simulink model "model_base"  (R2017b)
settings: Solver=VariableStepAuto  StartTime=0.0  StopTime=tfinal  MaxStep=0.1  RelTol=1e-9
values from neighbouring files (symbols this model uses):
  a = param.a    [EOM.m]    (also in KF_EOM.m; parameters.m = 1.08; roadPreview.m = obj.param.a; steadyState_EOM.m)
  a1 = obj.param.a1    [MPC.m]    (also in MPC_constraint.m = 0; RMPC.m; parameters.m = 0)
  a2 = obj.param.a2    [MPC.m]    (also in MPC_constraint.m = 1800; RMPC.m; parameters.m = 1800)
  a3 = obj.param.a3    [MPC.m]    (also in MPC_constraint.m = 100; RMPC.m; parameters.m = 100)
  a4 = obj.param.a4    [MPC.m]    (also in MPC_constraint.m = -100; RMPC.m; parameters.m = -100)
  a5 = obj.param.a5    [MPC.m]    (also in MPC_constraint.m = -1800; RMPC.m; parameters.m = -1800)
  A_road = sqrt(2*P*Dn)    [parameters.m]    (also in roadPreview.m = obj.param.A_road)
  b = param.b    [EOM.m]    (also in KF_EOM.m; parameters.m = 1.35; roadPreview.m = obj.param.b; spring.m = [0 (-ones(1,2*ne)).^j 0])
  B = param.B    [EOM.m]    (also in KF_EOM.m; MPC_EOM.m; RMPC.m = obj.param.B; parameters.m = 7.1)
  b1 = obj.param.b1    [MPC.m]    (also in MPC_constraint.m = 7500; RMPC.m; parameters.m = 7500)
  b2 = obj.param.b2    [MPC.m]    (also in MPC_constraint.m = 3000; RMPC.m; parameters.m = 3000)
  b3 = obj.param.b3    [MPC.m]    (also in MPC_constraint.m = 1666.66666667; RMPC.m; parameters.m = 1666.66666667)
  b4 = obj.param.b4    [MPC.m]    (also in MPC_constraint.m = 1666.66666667; RMPC.m; parameters.m = 1666.66666667)
  b5 = obj.param.b5    [MPC.m]    (also in MPC_constraint.m = 3000; RMPC.m; parameters.m = 3000)
  bcF = 2*zetac*omegasF*mF    (= 0)    [parameters.m]
  bcR = 2*zetac*omegasR*mR    (= 0)    [parameters.m]
  brake_init = [0; 0; 0; 0; x0]    [main.m]
  bsF = param.bsF    [EOM.m]    (also in KF_EOM.m; parameters.m = 3825.76172037; steadyState_EOM.m)
  bsR = param.bsR    [EOM.m]    (also in KF_EOM.m; parameters.m = 3672.73125156; steadyState_EOM.m)
  bt = param.bt    [EOM.m]    (also in KF_EOM.m; parameters.m = 0; steadyState_EOM.m)
  C = param.C    [EOM.m]    (also in KF_EOM.m; MPC_EOM.m; RMPC.m = obj.param.C; buildRoadFromPSD.m = 1e-06)
  Ccal = 1/kcal    (= 2.98507462687e-08)    [parameters.m]
  Ccyl = V0_brake/bhf    (= 1.88235294118e-14)    [parameters.m]
  D = param.D    [EOM.m]    (also in KF_EOM.m; MPC_EOM.m; RMPC.m = obj.param.D; parameters.m = 0.5)
  d_bump = 5    [parameters.m]    (also in roadPreview.m = obj.param.d_bump)
  g = param.g    [EOM.m]    (also in KF_EOM.m; MPC_EOM.m; RMPC.m = obj.param.g; parameters.m = 9.81)
  GcF_noInt = minreal(tf('s')*GcF)    [main.m]
  GcR_noInt = minreal(tf('s')*GcR)    [main.m]
  h_susp = param.h_susp    [EOM.m]    (also in KF_EOM.m; parameters.m = 0.2; steadyState_EOM.m)
  Icyl = mcyl    (= 0.75)    [parameters.m]
  Iline = phf*lline/(pi*dline^2/4)    (= 294259805.894)    [parameters.m]
  J = param.J    [EOM.m]    (also in KF_EOM.m; parameters.m = 1398.222; steadyState_EOM.m)
  Jw = param.Jw    [EOM.m]    (also in KF_EOM.m; MPC_EOM.m; RMPC.m = obj.param.Jw; parameters.m = 0.9)
  kcal = 3.35e7    (= 33500000)    [parameters.m]
  ksF = param.ksF    [EOM.m]    (also in KF_EOM.m; parameters.m = 30047.4622878; steadyState_EOM.m)
  ksR = param.ksR    [EOM.m]    (also in KF_EOM.m; parameters.m = 34614.6765555; steadyState_EOM.m)
  kt = param.kt    [EOM.m]    (also in KF_EOM.m; MPC_EOM.m; RMPC.m = obj.param.kt; parameters.m = 355305.758439)
  lambda_road = 50/3.6    (= 13.8888888889)    [parameters.m]    (also in roadPreview.m = obj.param.lambda_road)
  m = param.m    [EOM.m]    (also in KF_EOM.m; RMPC.m = [-ulb; uub]; parameters.m = 1370; steadyState_EOM.m)
  mF = param.mF    [EOM.m]    (also in KF_EOM.m; parameters.m = 761.111111111; steadyState_EOM.m)
  mR = param.mR    [EOM.m]    (also in KF_EOM.m; parameters.m = 608.888888889; steadyState_EOM.m)
  mucal = 0.4    [parameters.m]
  mus = param.mus    [EOM.m]    (also in KF_EOM.m; MPC.m = obj.param.mus; MPC_EOM.m; MPC_constraint.m)
  n_road = nmin:Dn:nmax    [parameters.m]    (also in roadPreview.m = obj.param.n_road)
  Phase_road = 2*pi*rand(size(A_road))    [parameters.m]    (also in roadPreview.m = obj.param.Phase_road)
  Rcyl = bcyl    (= 2500)    [parameters.m]
  reff = 0.112    [parameters.m]
  Rline = 128*phf*vhf*lline/(pi*dline^4)    (= 31387712628.7)    [parameters.m]
  roadProfile_index = 3    [getRoadIndex.m]    (also in main.m = getRoadIndex(roadProfile_name); roadPreview.m = obj.param.roadProfile_index)
  rw = param.rw    [EOM.m]    (also in KF_EOM.m; MPC_EOM.m; RMPC.m = obj.param.rw; parameters.m = 0.3)
  SAcyl = pi*dcyl^2/4    (= 0.00255175863288)    [parameters.m]
  state_init = [0 ... (first row only)    [main.m]
  sx_ref = -0.3    [MPC.m]    (also in RMPC.m; main.m = -1/B*tan(pi/(2*C)))
  sxABSoff = 0.1*sx_ref    [main.m]
  sxABSon_F = 1.4*sx_ref    [main.m]
  torque_request = -3000    [main.m]
  Ts_MPC = 0.05    [main.m]    (also in roadPreview.m = 0.01)
  U_cutoff = 10/3.6    (= 2.77777777778)    [main.m]
  w_road = 2*2*pi/lambda_road    (= 0.904778684234)    [parameters.m]    (also in roadPreview.m = obj.param.w_road)
  x0 = 0.00015    [parameters.m]    (also in test_minmaxMPC.m = rand(Nx,1))
  z0_road = 0.03    [parameters.m]    (also in roadPreview.m = obj.param.z0_road)
libraries: simulink x1
settings Model: Creator=louis  LastModifiedBy=louis

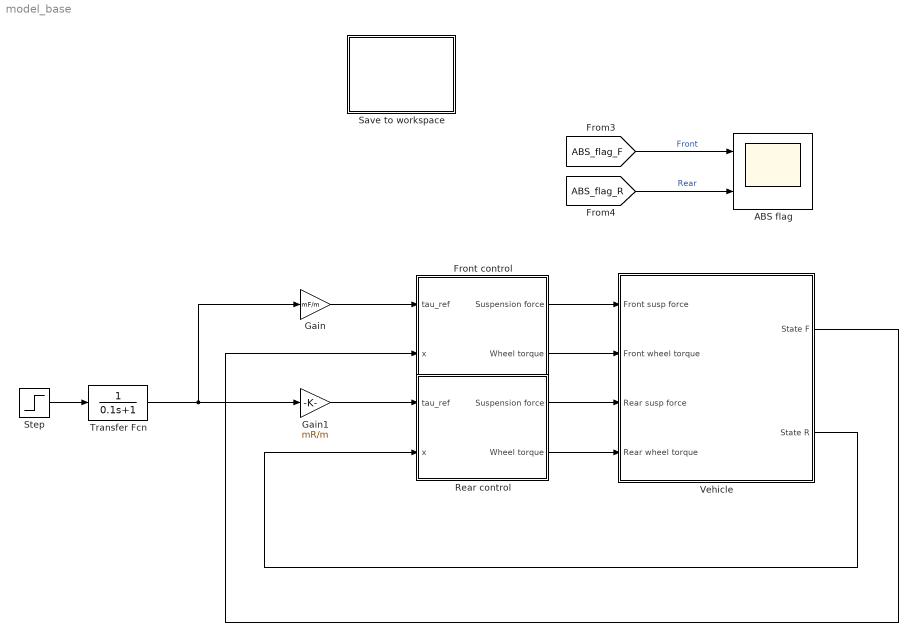
== system model_base ==
  ABS flag : Scope  NumInputPorts=2
  Front control : Subsystem
  Gain : Gain  Gain=mF/m
  Gain1 : Gain  Gain=mR/m
  Rear control : Subsystem
  Save to workspace : Subsystem
  Step : Step  After=torque_request  SampleTime=0
  Transfer Fcn : TransferFcn  Denominator=[0.1 1]
  Vehicle : Subsystem
  wires:
  Step/1 -> Transfer Fcn/1
  Transfer Fcn/1 -> Gain/1, Gain1/1
  Rear control/2(Wheel torque) -> Vehicle/4(Rear wheel torque)
  Vehicle/1(State F) -> Front control/2(x)
  Vehicle/2(State R) -> Rear control/2(x)
  Front control/2(Wheel torque) -> Vehicle/2(Front wheel torque)
  [ABS_flag_F] -> ABS flag/1  "Front"
  [ABS_flag_R] -> ABS flag/2  "Rear"
  Gain/1 -> Front control/1(tau_ref)
  Gain1/1 -> Rear control/1(tau_ref)
  Rear control/1(Suspension force) -> Vehicle/3(Rear susp force)
  Front control/1(Suspension force) -> Vehicle/1(Front susp force)

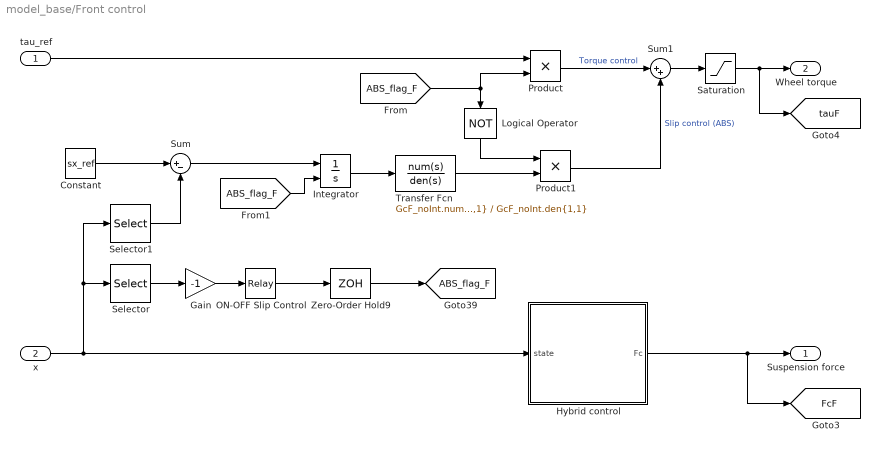
== system model_base/Front control ==
  tau_ref : Inport
  x : Inport  Port=2
  Constant : Constant  Value=sx_ref
  Gain : Gain  Gain=-1
  Hybrid control : MATLAB Function  TreatAsAtomicUnit=on
  Integrator : Integrator  ExternalReset=rising
  Logical Operator : Logic  Operator=NOT  AllPortsSameDT=off  OutDataTypeStr=boolean
  ON-OFF Slip Control : Relay  OnSwitchValue=-sxABSon_F  OffSwitchValue=-sxABSoff  OnOutputValue=0  OffOutputValue=1
  Product : Product
  Product1 : Product
  Saturation : Saturate  UpperLimit=0  LowerLimit=-Inf
  Selector : Selector  IndexOptions=Index vector (dialog)  Indices=5  OutputSizes=1
  Selector1 : Selector  IndexOptions=Index vector (dialog)  Indices=5  OutputSizes=1
  Sum : Sum  Inputs=|+-
  Sum1 : Sum  Inputs=|++
  Transfer Fcn : TransferFcn  Numerator=GcF_noInt.num{1,1}  Denominator=GcF_noInt.den{1,1}
  Zero-Order Hold9 : ZeroOrderHold  SampleTime=Ts_MPC
  Suspension force : Outport
  Wheel torque : Outport  Port=2
  tag scope: ABS_flag_F=global, FcF=global, tauF=global
  wires:
  x/1 -> Hybrid control/1(state), Selector1/1, Selector/1
  Zero-Order Hold9/1 -> [ABS_flag_F]
  Gain/1 -> ON-OFF Slip Control/1
  Selector/1 -> Gain/1
  ON-OFF Slip Control/1 -> Zero-Order Hold9/1
  tau_ref/1 -> Product/1
  Sum1/1 -> Saturation/1
  Hybrid control/1(Fc) -> [FcF], Suspension force/1
  Integrator/1 -> Transfer Fcn/1
  [ABS_flag_F] -> Product/2, Logical Operator/1
  Logical Operator/1 -> Product1/1
  Constant/1 -> Sum/1
  Transfer Fcn/1 -> Product1/2
  [ABS_flag_F] -> Integrator/2
  Sum/1 -> Integrator/1
  Selector1/1 -> Sum/2
  Product/1 -> Sum1/1  "Torque control"
  Product1/1 -> Sum1/2  "Slip control (ABS)"
  Saturation/1 -> [tauF], Wheel torque/1

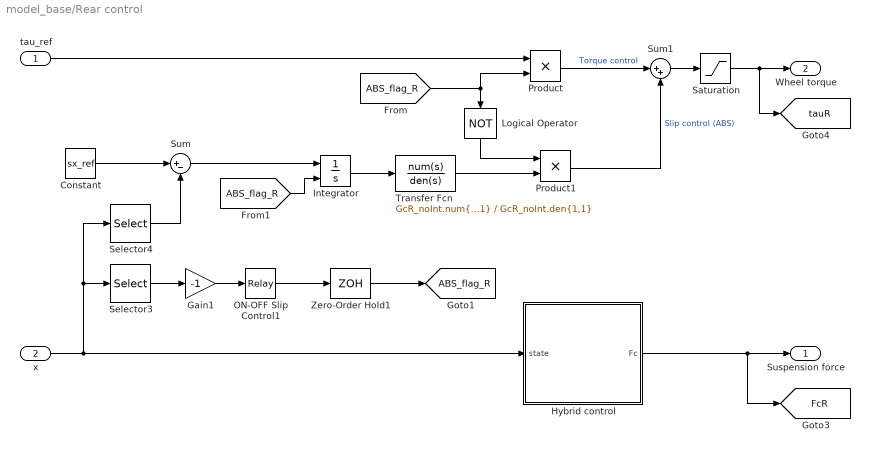
== system model_base/Rear control ==
  tau_ref : Inport
  x : Inport  Port=2
  Constant : Constant  Value=sx_ref
  Gain1 : Gain  Gain=-1
  Hybrid control : MATLAB Function  TreatAsAtomicUnit=on
  Integrator : Integrator  ExternalReset=either
  Logical Operator : Logic  Operator=NOT  AllPortsSameDT=off  OutDataTypeStr=boolean
  ON-OFF Slip Control1 : Relay  OnSwitchValue=-sxABSon_F  OffSwitchValue=-sxABSoff  OnOutputValue=0  OffOutputValue=1
  Product : Product
  Product1 : Product
  Saturation : Saturate  UpperLimit=0  LowerLimit=-Inf
  Selector3 : Selector  IndexOptions=Index vector (dialog)  Indices=5  OutputSizes=1
  Selector4 : Selector  IndexOptions=Index vector (dialog)  Indices=5  OutputSizes=1
  Sum : Sum  Inputs=|+-
  Sum1 : Sum  Inputs=|++
  Transfer Fcn : TransferFcn  Numerator=GcR_noInt.num{1,1}  Denominator=GcR_noInt.den{1,1}
  Zero-Order Hold1 : ZeroOrderHold  SampleTime=Ts_MPC
  Suspension force : Outport
  Wheel torque : Outport  Port=2
  tag scope: ABS_flag_R=global, FcR=global, tauR=global
  wires:
  ON-OFF Slip Control1/1 -> Zero-Order Hold1/1
  Selector3/1 -> Gain1/1
  Zero-Order Hold1/1 -> [ABS_flag_R]
  Sum1/1 -> Saturation/1
  tau_ref/1 -> Product/1
  Product1/1 -> Sum1/2  "Slip control (ABS)"
  Gain1/1 -> ON-OFF Slip Control1/1
  Logical Operator/1 -> Product1/1
  [ABS_flag_R] -> Integrator/2
  Constant/1 -> Sum/1
  Hybrid control/1(Fc) -> [FcR], Suspension force/1
  Product/1 -> Sum1/1  "Torque control"
  Integrator/1 -> Transfer Fcn/1
  [ABS_flag_R] -> Product/2, Logical Operator/1
  Selector4/1 -> Sum/2
  x/1 -> Hybrid control/1(state), Selector4/1, Selector3/1
  Sum/1 -> Integrator/1
  Transfer Fcn/1 -> Product1/2
  Saturation/1 -> [tauR], Wheel torque/1

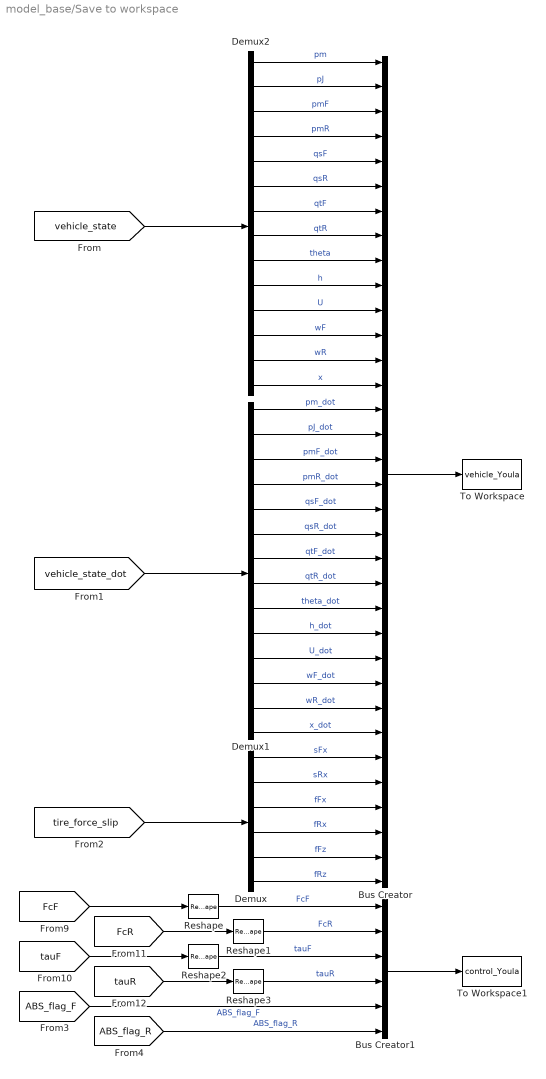
== system model_base/Save to workspace ==
  Bus Creator : BusCreator  Inputs=34
  Bus Creator1 : BusCreator  Inputs=6
  Demux : Demux  Outputs=6
  Demux1 : Demux  Outputs=14
  Demux2 : Demux  Outputs=14
  Reshape{,1..3} (4 alike) : Reshape
  To Workspace : ToWorkspace  VariableName=vehicle_Youla  SaveFormat=Timeseries  SampleTime=-1
  To Workspace1 : ToWorkspace  VariableName=control_Youla  SaveFormat=Timeseries  SampleTime=-1
  wires:
  Demux/1 -> Bus Creator/29  "sFx"
  [tire_force_slip] -> Demux/1
  Demux/2 -> Bus Creator/30  "sRx"
  Demux/3 -> Bus Creator/31  "fFx"
  Demux/5 -> Bus Creator/33  "fFz"
  [vehicle_state] -> Demux2/1
  Bus Creator/1 -> To Workspace/1
  Demux2/1 -> Bus Creator/1  "pm"
  Demux2/2 -> Bus Creator/2  "pJ"
  Demux2/3 -> Bus Creator/3  "pmF"
  Demux2/4 -> Bus Creator/4  "pmR"
  Demux2/5 -> Bus Creator/5  "qsF"
  Demux2/6 -> Bus Creator/6  "qsR"
  Demux2/7 -> Bus Creator/7  "qtF"
  Demux2/8 -> Bus Creator/8  "qtR"
  Demux2/9 -> Bus Creator/9  "theta"
  Demux2/11 -> Bus Creator/11  "U"
  Demux2/12 -> Bus Creator/12  "wF"
  Demux2/13 -> Bus Creator/13  "wR"
  Demux2/14 -> Bus Creator/14  "x"
  Demux/6 -> Bus Creator/34  "fRz"
  Demux/4 -> Bus Creator/32  "fRx"
  Demux1/2 -> Bus Creator/16  "pJ_dot"
  Demux1/11 -> Bus Creator/25  "U_dot"
  Demux1/8 -> Bus Creator/22  "qtR_dot"
  Demux1/4 -> Bus Creator/18  "pmR_dot"
  Demux1/5 -> Bus Creator/19  "qsF_dot"
  Demux1/9 -> Bus Creator/23  "theta_dot"
  Demux1/14 -> Bus Creator/28  "x_dot"
  Demux1/1 -> Bus Creator/15  "pm_dot"
  Demux1/13 -> Bus Creator/27  "wR_dot"
  Demux1/7 -> Bus Creator/21  "qtF_dot"
  [vehicle_state_dot] -> Demux1/1
  Demux1/3 -> Bus Creator/17  "pmF_dot"
  Demux1/12 -> Bus Creator/26  "wF_dot"
  Demux1/6 -> Bus Creator/20  "qsR_dot"
  Demux2/10 -> Bus Creator/10  "h"
  Demux1/10 -> Bus Creator/24  "h_dot"
  [ABS_flag_F] -> Bus Creator1/5  "ABS_flag_F"
  [ABS_flag_R] -> Bus Creator1/6  "ABS_flag_R"
  Bus Creator1/1 -> To Workspace1/1
  Reshape1/1 -> Bus Creator1/2  "FcR"
  Reshape/1 -> Bus Creator1/1  "FcF"
  Reshape3/1 -> Bus Creator1/4  "tauR"
  Reshape2/1 -> Bus Creator1/3  "tauF"
  [FcF] -> Reshape/1
  [FcR] -> Reshape1/1
  [tauF] -> Reshape2/1
  [tauR] -> Reshape3/1

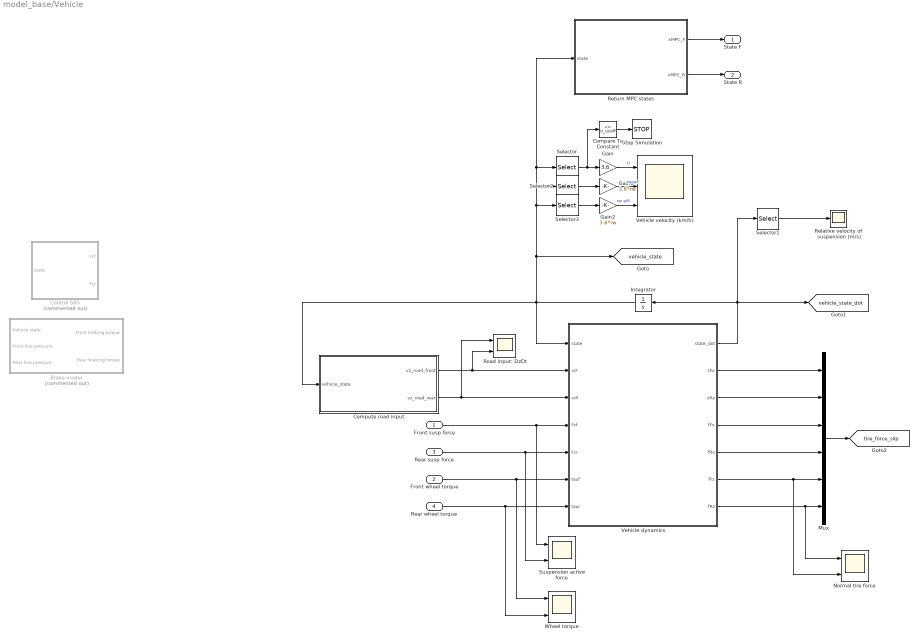
== system model_base/Vehicle ==
  Front susp force : Inport
  Front wheel torque : Inport  Port=2
  Rear susp force : Inport  Port=3
  Rear wheel torque : Inport  Port=4
  Brake model : Subsystem  Commented=on
  Compare To Constant : simulink/Logic and Bit Operations/Compare To Constant  relop=<=  const=U_cutoff  OutDataTypeStr=boolean
  Compute road input : MATLAB Function  TreatAsAtomicUnit=on
  Control SAS : MATLAB Function  Commented=on  TreatAsAtomicUnit=on
  Gain : Gain  Gain=3.6
  Gain1 : Gain  Gain=3.6*rw
  Gain2 : Gain  Gain=3.6*rw
  Integrator : Integrator  InitialCondition=state_init
  Mux : Mux  Inputs=6
  Normal tire force : Scope  NumInputPorts=2
  Relative velocity of suspension (m/s) : Scope
  Return MPC states : MATLAB Function  TreatAsAtomicUnit=on
  Road input: DzDt : Scope  NumInputPorts=2
  Selector : Selector  IndexOptions=Index vector (dialog)  Indices=11  OutputSizes=1
  Selector1 : Selector  IndexOptions=Index vector (dialog)  Indices=[5 6]  OutputSizes=1
  Selector2 : Selector  IndexOptions=Index vector (dialog)  Indices=12  OutputSizes=1
  Selector3 : Selector  IndexOptions=Index vector (dialog)  Indices=13  OutputSizes=1
  Stop Simulation : Stop
  Suspension active force : Scope  NumInputPorts=2
  Vehicle dynamics : MATLAB Function  TreatAsAtomicUnit=on
  Vehicle velocity (km/h) : Scope  NumInputPorts=3
  Wheel torque : Scope  NumInputPorts=2
  State F : Outport
  State R : Outport  Port=2
  tag scope: tire_force_slip=global, vehicle_state=global, vehicle_state_dot=global
  wires:
  Gain/1 -> Vehicle velocity (km/h)/1  "U"
  Vehicle dynamics/7(fRz) -> Normal tire force/1, Mux/6
  Vehicle dynamics/3(sRx) -> Mux/2
  Vehicle dynamics/4(fFx) -> Mux/3
  Vehicle dynamics/5(fRx) -> Mux/4
  Selector/1 -> Compare To Constant/1, Gain/1
  Vehicle dynamics/2(sFx) -> Mux/1
  Vehicle dynamics/1(state_dot) -> Integrator/1, Selector1/1, [vehicle_state_dot]
  Vehicle dynamics/6(fFz) -> Normal tire force/2, Mux/5
  Mux/1 -> [tire_force_slip]
  Compute road input/2(vz_road_rear) -> Vehicle dynamics/3(viR), Road input: DzDt/1
  Front wheel torque/1 -> Wheel torque/1, Vehicle dynamics/6(tauf)
  Rear wheel torque/1 -> Wheel torque/2, Vehicle dynamics/7(taur)
  Compare To Constant/1 -> Stop Simulation/1
  Front susp force/1 -> Suspension active force/1, Vehicle dynamics/4(Fcf)
  Rear susp force/1 -> Suspension active force/2, Vehicle dynamics/5(Fcr)
  Compute road input/1(vz_road_front) -> Vehicle dynamics/2(viF), Road input: DzDt/2
  Selector1/1 -> Relative velocity of suspension (m/s)/1
  Integrator/1 -> Vehicle dynamics/1(state), [vehicle_state], Selector3/1, Selector2/1, Return MPC states/1(state), Selector/1, Compute road input/1(vehicle_state)
  Return MPC states/1(xMPC_F) -> State F/1
  Return MPC states/2(xMPC_R) -> State R/1
  Selector2/1 -> Gain1/1
  Gain1/1 -> Vehicle velocity (km/h)/2  "rw wF"
  Gain2/1 -> Vehicle velocity (km/h)/3  "rw wR"
  Selector3/1 -> Gain2/1

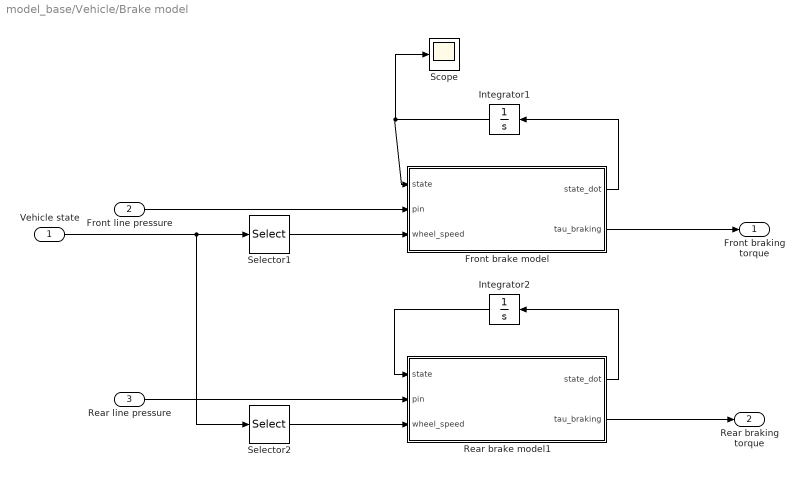
== system model_base/Vehicle/Brake model ==
  Vehicle state : Inport
  Front line pressure : Inport  Port=2
  Rear line pressure : Inport  Port=3
  Front brake model : MATLAB Function  TreatAsAtomicUnit=on
  Integrator1 : Integrator  InitialCondition=brake_init
  Integrator2 : Integrator  InitialCondition=brake_init
  Rear brake model1 : MATLAB Function  TreatAsAtomicUnit=on
  Scope : Scope
  Selector1 : Selector  IndexOptions=Index vector (dialog)  Indices=12  OutputSizes=1
  Selector2 : Selector  IndexOptions=Index vector (dialog)  Indices=13  OutputSizes=1
  Front braking torque : Outport
  Rear braking torque : Outport  Port=2
  wires:
  Front brake model/1(state_dot) -> Integrator1/1
  Vehicle state/1 -> Selector2/1, Selector1/1
  Integrator1/1 -> Scope/1, Front brake model/1(state)
  Front brake model/2(tau_braking) -> Front braking torque/1
  Selector1/1 -> Front brake model/3(wheel_speed)
  Front line pressure/1 -> Front brake model/2(pin)
  Selector2/1 -> Rear brake model1/3(wheel_speed)
  Rear line pressure/1 -> Rear brake model1/2(pin)
  Integrator2/1 -> Rear brake model1/1(state)
  Rear brake model1/1(state_dot) -> Integrator2/1
  Rear brake model1/2(tau_braking) -> Rear braking torque/1

== matlab function model_base/Vehicle/Compute road input ==
  data: vz_road_front output; vehicle_state input; vz_road_rear output; a parameter; b parameter; J parameter; z0_road parameter; w_road parameter; lambda_road parameter; d_bump parameter; A_road parameter; Phase_road parameter; n_road parameter; roadProfile_index parameter
function [vz_road_front,vz_road_rear] = roadInput(vehicle_state, ...
    a, b, J, z0_road, w_road, lambda_road, d_bump,...
    A_road, Phase_road, n_road, roadProfile_index)

pJ    = vehicle_state(2);
theta = vehicle_state(9);
U     = vehicle_state(11);
x     = vehicle_state(14);
theta_dot = pJ/J;
x_dot     = U;

% Compute longitudinal speed at front and rear wheel
x_front = x + a*cos(theta);
x_rear  = x - b*cos(theta);
DxDt_front = x_dot - a*theta_dot*sin(theta);
DxDt_rear  = x_dot + b*theta_dot*sin(theta);

% Road input at the front wheel is:
% x_dot - a*theta_dot*sin(theta) * dz_road/dx(x -b cos(theta))
DzDx_front = roadProfile(x_front,z0_road,lambda_road,w_road,d_bump,...
    A_road,Phase_road,n_road,roadProfile_index);
vz_road_front = DxDt_front * DzDx_front;

% Road input at the rear wheel is:
% x_dot + b*theta_dot*sin(theta) * dz_road/dx(x -b cos(theta))
DzDx_rear = roadProfile(x_rear,z0_road,lambda_road,w_road,d_bump,...
    A_road,Phase_road,n_road,roadProfile_index);
vz_road_rear = DxDt_rear * DzDx_rear;

== matlab function model_base/Vehicle/Vehicle dynamics ==
  data: state input; viF input; state_dot output; sFx output; sRx output; fFx output; fRx output; fFz output; fRz output; viR input; Fcf input; Fcr input; tauf input; taur input; m parameter; J parameter; a parameter; b parameter; ksR parameter; ksF parameter; bsR parameter; bsF parameter; kt parameter; bt parameter; mus parameter; rw parameter; B parameter; C parameter; D parameter; Jw parameter; g parameter; h_susp parameter; mF parameter; mR parameter
function [state_dot,sFx,sRx,fFx,fRx,fFz,fRz] = ...
    chassisModel(state,viF,viR,Fcf, Fcr,tauf,taur,...
    m, J, a, b, ksR, ksF, bsR, bsF, kt, bt, mus, rw, B, C, D, Jw, g, ...
    h_susp, mF, mR)

%% Rename state variables
% Vertical dynamics
pm    = state(1);
pJ    = state(2);
pmF   = state(3);
pmR   = state(4);
qsF   = state(5);
qsR   = state(6);
qtF   = state(7);
qtR   = state(8);
theta = state(9);
% h     = state(10);
% Longitudinal dynamics
U     = state(11);
wF    = state(12);
wR    = state(13);
% x     = state(14);

% Compute vertical velocities at the front and rear of the sprung mass
vR  = pm/m - b*cos(theta) * pJ/J;
vF  = pm/m + a*cos(theta) * pJ/J;

% Compute distance
h_susp_F = h_susp - qsF;            % Height of the front suspension
h_susp_R = h_susp - qsR;            % Height of the rear suspension
rwF_unladen = rw + (mF+mus)*g/kt;   % Unladen front wheel radius
rwR_unladen = rw + (mR+mus)*g/kt;   % Unladen rear wheel radius
rwF = min(rw - qtF, rwF_unladen);   % Front tire radius
rwR = min(rw - qtR, rwR_unladen);   % Rear tire radius

%% Compute suspension and tire forces
% Suspension vertical forces (gauge)
fsF = ksF*qsF + Fcf + bsF*(pmF/mus - vF);
fsR = ksR*qsR + Fcr + bsR*(pmR/mus - vR);

% data = [ -1410, -5008;
%  -720, -3436;
%  -390, -2324;
%  -210, -1792;
%  -90, -1008;
%  -20, -228;
%  20, 228;
%  90, 596;
%  200, 784;
%  390, 1100;
%  760, 1796;
%  1160, 2560];
% v_rel = data(:,1)*1e-3; % Relative velocity (m/s)
% F_damper = 2*data(:,2); % Damper force for one axle (N)
% % TODO check sign: 
% % is it interp1(v_rel,-F_damper,-(pmF/mus - vF),'linear','extrap')
% % or interp1(v_rel,F_damper,(pmF/mus - vF),'linear','extrap')
% F_damper_F = interp1(v_rel,-F_damper,-(pmF/mus - vF),'linear','extrap');
% F_damper_R = interp1(v_rel,-F_damper,-(pmR/mus - vR),'linear','extrap');
% fsF = ksF*qsF + Fcf + F_damper_F;
% fsR = ksR*qsR + Fcr + F_damper_R;

% Tire vertical forces (gauge)
ftF = kt*qtF + bt*(viF - pmF/mus);
ftR = kt*qtR + bt*(viR - pmR/mus);

% Make sure the tire vertical force cannot be negative
ftF = max(-(mus + mF)*g,ftF);
ftR = max(-(mus + mR)*g,ftR);

%% Compute longitudinal tire force
% Compute longitudinal slip ratio
% Front slip ratio
den = max(rwF * wF, U);
if den ~= 0
    sFx = (rwF * wF - U) / den;
else
    sFx = 0;
end
% Rear slip ratio
den = max(rwR * wR, U);
if den ~= 0
    sRx = (rwR * wR - U) / den;
else
    sRx = 0;
end

% Compute friction coefficient (simplified Pacejka's tire model)
muF = D * sin(C * atan(B * sFx));
muR = D * sin(C * atan(B * sRx));

% Compute normal force
fFz = ftF + (mus + mF)*g;
fRz = ftR + (mus + mR)*g;

% Compute longitudinal force
fFx = fFz * muF;
fRx = fRz * muR;


%% Compute the state derivatives
% Vertical dynamics
pm_dot    = fsR + fsF;
pJ_dot    = a*cos(theta) * fsF - b*cos(theta) * fsR ...
          + (h_susp_F + rwF - a*sin(theta)) * fFx ...
          + (h_susp_R + rwR + b*sin(theta)) * fRx;
pmF_dot   = ftF - fsF;
pmR_dot   = ftR - fsR;
qsF_dot   = pmF/mus - vF;
qsR_dot   = pmR/mus - vR;
qtF_dot   = viF - pmF/mus;
qtR_dot   = viR - pmR/mus;
theta_dot = pJ/J;
h_dot     = pm/m;

% Longitudinal dynamics
U_dot = 1/(m+2*mus) * (fFx + fRx);
wF_dot = 1/Jw * (tauf - rwF*fFx);
wR_dot = 1/Jw * (taur - rwR*fRx);
x_dot = U;

%% Return the state derivatives
state_dot = [pm_dot; pJ_dot; pmF_dot; pmR_dot;...
    qsF_dot; qsR_dot; qtF_dot; qtR_dot; theta_dot; h_dot;...
    U_dot; wF_dot; wR_dot; x_dot];

end

== matlab function model_base/Vehicle/Brake model/Front brake model ==
  data: state input; state_dot output; pin input; wheel_speed input; tau_braking output; Icyl parameter; Rcyl parameter; Ccal parameter; Iline parameter; Rline parameter; Ccyl parameter; SAcyl parameter; mucal parameter; kcal parameter; reff parameter; x0 parameter
function [state_dot, tau_braking] = brakeModel(state, pin, wheel_speed, ...
    Icyl, Rcyl, Ccal, Iline, Rline, Ccyl, SAcyl, mucal, kcal, reff, x0)

%% Rename state variables
pline = state(1);
qcyl  = state(2);
pcyl  = state(3);
qcal  = state(4);
xcal  = state(5);

%% Equation of motion
pline_dot = pin - Rline*pline/Iline - qcyl/Ccyl;
qcyl_dot  = pline/Iline - SAcyl*pcyl/Icyl;
pcyl_dot  = SAcyl*qcyl/Ccyl - Rcyl*pcyl/Icyl - qcal/Ccal;
qcal_dot  = pcyl/Icyl;
xcal_dot  = pcyl/Icyl;

%% Pack state derivatives
state_dot = [pline_dot; qcyl_dot; pcyl_dot; qcal_dot; xcal_dot];

%% Compute braking torque
tau_braking = 2*mucal*reff*kcal * max(xcal - x0, 0);
% Braking torque is always in the opposite direction to the wheelspeed
tau_braking = -tau_braking * sign(wheel_speed);

== matlab function model_base/Vehicle/Brake model/Rear brake model1 ==
  data: state input; state_dot output; pin input; wheel_speed input; tau_braking output; Icyl parameter; Rcyl parameter; Ccal parameter; Iline parameter; Rline parameter; Ccyl parameter; SAcyl parameter; mucal parameter; kcal parameter; reff parameter; x0 parameter
function [state_dot, tau_braking] = brakeModel(state, pin, wheel_speed, ...
    Icyl, Rcyl, Ccal, Iline, Rline, Ccyl, SAcyl, mucal, kcal, reff, x0)

%% Rename state variables
pline = state(1);
qcyl  = state(2);
pcyl  = state(3);
qcal  = state(4);
xcal  = state(5);

%% Equation of motion
pline_dot = pin - Rline*pline/Iline - qcyl/Ccyl;
qcyl_dot  = pline/Iline - SAcyl*pcyl/Icyl;
pcyl_dot  = SAcyl*qcyl/Ccyl - Rcyl*pcyl/Icyl - qcal/Ccal;
qcal_dot  = pcyl/Icyl;
xcal_dot  = pcyl/Icyl;

%% Pack state derivatives
state_dot = [pline_dot; qcyl_dot; pcyl_dot; qcal_dot; xcal_dot];

%% Compute braking torque
tau_braking = 2*mucal*reff*kcal * max(xcal - x0, 0);
% Braking torque is always in the opposite direction to the wheelspeed
tau_braking = -tau_braking * sign(wheel_speed);

== matlab function model_base/Vehicle/Control SAS ==
  data: Fcf output; Fcr output; state input; m parameter; a parameter; b parameter; J parameter; bcF parameter; bcR parameter; mus parameter
function [Fcf,Fcr] = controlSAS(state,m, a, b, J, bcF, bcR, mus)

pm    = state(1);
pJ    = state(2);
pmF   = state(3);
pmR   = state(4);
theta = state(9);

vF  = pm/m + a*cos(theta) * pJ/J;
vR  = pm/m - b*cos(theta) * pJ/J;

Fcr = -bcR * vR;
if Fcr * (pmR/mus - vR) < 0
    Fcr = 0;
end
Fcf = -bcF * vF;
if Fcf * (pmF/mus - vF) < 0
    Fcf = 0;
end

== matlab function model_base/Front control/Hybrid control ==
  data: state input; Fc output; mF parameter; mus parameter; a1 parameter; a2 parameter; a3 parameter; a4 parameter; a5 parameter; b1 parameter; b2 parameter; b3 parameter; b4 parameter; b5 parameter
function Fc = hybridControl(state,mF, mus, a1, a2, a3, a4, a5,...
b1, b2, b3, b4, b5)

% Rename states
pspr = state(1);
puns = state(2);

% Found bounds on the suspension
msp = mF;
vrel = -(pspr/msp - puns/mus);
vm = (a1-a4) / (b4-b1);
vp = (a1-a3) / (b3-b1);
if vrel < vm
    Fcmin = max(b1 * vrel + a1, b5 * vrel + a5);
    Fcmax = (b4 * vrel + a4);
elseif vrel <= vp
    Fcmin = (b1 * vrel + a1);
    Fcmax = (b1 * vrel + a1);
else
    Fcmin = (b3 * vrel + a3);
    Fcmax = min(b1 * vrel + a1, b2 * vrel + a2);
end

% Use hybrid control strategy
qs_dot = puns/mus - pspr/msp;
if pspr*qs_dot <= 0
    Fc = Fcmin;
else
    Fc = Fcmax;
end

== matlab function model_base/Rear control/Hybrid control ==
  data: state input; Fc output; mR parameter; mus parameter; a1 parameter; a2 parameter; a3 parameter; a4 parameter; a5 parameter; b1 parameter; b2 parameter; b3 parameter; b4 parameter; b5 parameter
function Fc = hybridControl(state,mR, mus, a1, a2, a3, a4, a5,...
b1, b2, b3, b4, b5)

% Rename states
pspr = state(1);
puns = state(2);

% Found bounds on the suspension
msp = mR;
vrel = -(pspr/msp - puns/mus);
vm = (a1-a4) / (b4-b1);
vp = (a1-a3) / (b3-b1);
if vrel < vm
    Fcmin = max(b1 * vrel + a1, b5 * vrel + a5);
    Fcmax = (b4 * vrel + a4);
elseif vrel <= vp
    Fcmin = (b1 * vrel + a1);
    Fcmax = (b1 * vrel + a1);
else
    Fcmin = (b3 * vrel + a3);
    Fcmax = min(b1 * vrel + a1, b2 * vrel + a2);
end

% Use hybrid control strategy
qs_dot = puns/mus - pspr/msp;
if pspr*qs_dot <= 0
    Fc = Fcmin;
else
    Fc = Fcmax;
end

== matlab function model_base/Vehicle/Return MPC states ==
  data: state input; xMPC_F output; xMPC_R output; m parameter; a parameter; b parameter; J parameter; rw parameter; mF parameter; mR parameter; mus parameter; g parameter; kt parameter
function [xMPC_F, xMPC_R] = stateMPC(state, m, a, b, J, rw, mF, mR, ...
mus, g, kt)
% Return the state of the MPC

%% Unpack the states
% Vertical dynamics
pm    = state(1);
pJ    = state(2);
pmF   = state(3);
pmR   = state(4);
qsF   = state(5);
qsR   = state(6);
qtF   = state(7);
qtR   = state(8);
theta = state(9);
% h     = state(10);
% Longitudinal dynamics
U     = state(11);
wF    = state(12);
wR    = state(13);
% x     = state(14);

% Compute vertical velocities at the front and rear of the sprung mass
vR  = pm/m - b*cos(theta) * pJ/J;
vF  = pm/m + a*cos(theta) * pJ/J;

%% Compute the slip
rwF_unladen = rw + (mF+mus)*g/kt;   % Unladen front wheel radius
rwR_unladen = rw + (mR+mus)*g/kt;   % Unladen rear wheel radius
rwF = min(rw - qtF, rwF_unladen);   % Front tire radius
rwR = min(rw - qtR, rwR_unladen);   % Rear tire radius

% Front slip ratio
den = max(rwF * wF, U);
if den ~= 0
    sFx = (rwF * wF - U) / den;
else
    sFx = 0;
end
% Rear slip ratio
den = max(rwR * wR, U);
if den ~= 0
    sRx = (rwR * wR - U) / den;
else
    sRx = 0;
end

%% Return the MPC states
xMPC_F = [mF*vF; pmF; qsF; qtF; sFx];
xMPC_R = [mR*vR; pmR; qsR; qtR; sRx];
